simulink model "Motor_R2019a"  (R2019a)
settings: Solver=VariableStepAuto  StartTime=0.0  StopTime=10.0  RelTol=1e-3
model workspace (MAT data in the model file):
  Jm = 0.1
  Kb = 3
  Ki = 5
  L = 10
  R = 100
settings Model: Creator=Haier  LastModifiedBy=Haier

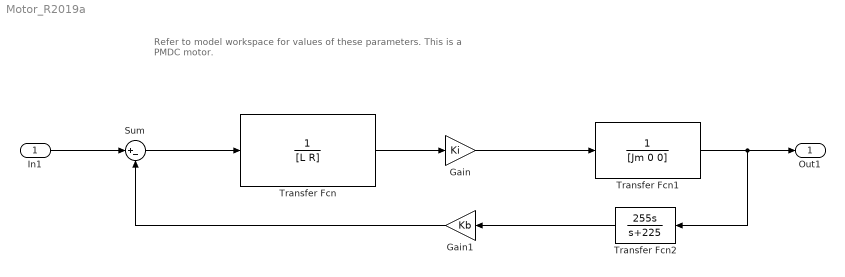
== system Motor_R2019a ==
  note: Refer to model workspace for values of these
      | parameters. This is a PMDC motor.
  In1 : Inport
  Gain : Gain  Gain=Ki
  Gain1 : Gain  Gain=Kb
  Sum : Sum  Inputs=|+-
  Transfer Fcn : TransferFcn  Denominator=[L R]
  Transfer Fcn1 : TransferFcn  Denominator=[Jm 0 0]
  Transfer Fcn2 : TransferFcn  Numerator=[255 0]  Denominator=[1 225]
  Out1 : Outport
  wires:
  In1/1 -> Sum/1
  Sum/1 -> Transfer Fcn/1
  Transfer Fcn/1 -> Gain/1
  Gain/1 -> Transfer Fcn1/1
  Transfer Fcn1/1 -> Transfer Fcn2/1, Out1/1
  Transfer Fcn2/1 -> Gain1/1
  Gain1/1 -> Sum/2
